simulink model "T10_LoNhiet"  (R2013b)
settings: Solver=ode5  StartTime=0.0  StopTime=inf  RelTol=1e-3
undefined symbols (not defined in the file or in its folder): National_Instruments, PCI
libraries: rtwinlib x4, dsparch4 x1, simulink x1
settings Model: SimulationMode=external  Creator=Administrator  LastModifiedBy=Administrator
settings HardwareCC: ProdIntDivRoundTo=Zero  ProdEndianess=LittleEndian  ProdHWDeviceType=Generic->32-bit x86 compatible
settings RTWCC: SystemTargetFile=rtwin.tlc  TemplateMakefile=rtwin.tmf  Description=Real-Time Windows Target  ProcessScript=rtwin_make_rtw_hook  RTWCompilerOptimization=On
settings CodeAppCC: MaxIdLength=95
settings RTWinTargetCC: TargetLibSuffix=_rtwin.lib  TargetPreCompLibLocation=C:\Program Files\MATLAB\R2013b\toolbox\rtw\targets\rtwin\lib\win64  CodeReplacementLibrary=ANSI_C  RTWinDir=C:/PROGRA~1/MATLAB/R2013b/toolbox/rtw/targets/rtwin  TargetArch=win64

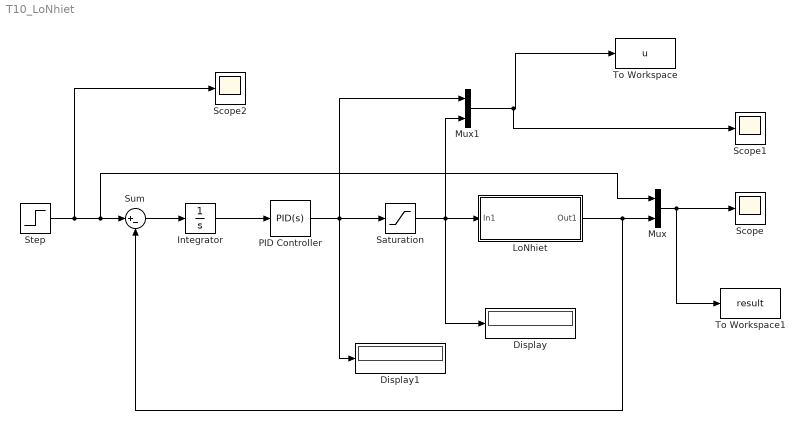
== system T10_LoNhiet ==
  Display : Display
  Display1 : Display
  Integrator : Integrator
  "LoNhiet " : Subsystem
  Mux : Mux  Inputs=2
  Mux1 : Mux  Inputs=2
  PID Controller : simulink/Continuous/PID Controller  Controller=PID  TimeDomain=Continuous-time  SampleTime=1  IntegratorMethod=Forward Euler  FilterMethod=Forward Euler  Form=Parallel  P=0.01  I=0.0005  D=0.0000025  N=100  InitialConditionSource=internal  InitialConditionForIntegrator=0  InitialConditionForFilter=0  ExternalReset=none  LimitOutput=off  UpperSaturationLimit=inf  LowerSaturationLimit=-inf  LinearizeAsGain=on  AntiWindupMode=none  Kb=1  TrackingMode=off  Kt=1  PParamMin=[]  PParamMax=[]  IParamMin=[]  IParamMax=[]  DParamMin=[]  DParamMax=[]  NParamMin=[]  NParamMax=[]  KbParamMin=[]  KbParamMax=[]  KtParamMin=[]  KtParamMax=[]  POutMin=[]  POutMax=[]  IOutMin=[]  IOutMax=[]  DOutMin=[]  DOutMax=[]  NOutMin=[]  NOutMax=[]  KbOutMin=[]  KbOutMax=[]  KtOutMin=[]  KtOutMax=[]  IntegratorOutMin=[]  IntegratorOutMax=[]  FilterOutMin=[]  FilterOutMax=[]  SumOutMin=[]  SumOutMax=[]  SumI1OutMin=[]  SumI1OutMax=[]  SumI2OutMin=[]  SumI2OutMax=[]  SumI3OutMin=[]  SumI3OutMax=[]  SumDOutMin=[]  SumDOutMax=[]  SaturationOutMin=[]  SaturationOutMax=[]  IntegratorContinuousStateAttributes=''  IntegratorStateMustResolveToSignalObject=off  IntegratorRTWStateStorageClass=Auto  FilterContinuousStateAttributes=''  FilterStateMustResolveToSignalObject=off  FilterRTWStateStorageClass=Auto
  Saturation : Saturate  UpperLimit=12  LowerLimit=0
  Scope : Scope
      settings: YMin=48  YMax=60
  Scope1 : Scope
      settings: YMin=0  YMax=2000
  Scope2 : Scope
      settings: YMin=60  YMax=60  SaveName=ScopeData2
  Step : Step  Time=0  After=60  SampleTime=0
  Sum : Sum  Inputs=|+-
  To Workspace : ToWorkspace  VariableName=u  SampleTime=-1  SaveFormat=Timeseries
  To Workspace1 : ToWorkspace  VariableName=result  SampleTime=-1  SaveFormat=Timeseries
  wires:
  Sum/1 -> Integrator/1
  Integrator/1 -> PID Controller/1
  PID Controller/1 -> Mux1/1, Display1/1, Saturation/1
  Saturation/1 -> Display/1, Mux1/2, "LoNhiet "/1(In1)
  Mux1/1 -> Scope1/1, To Workspace/1
  Mux/1 -> To Workspace1/1, Scope/1
  Step/1 -> Scope2/1, Mux/1, Sum/1
  "LoNhiet "/1(Out1) -> Sum/2, Mux/2

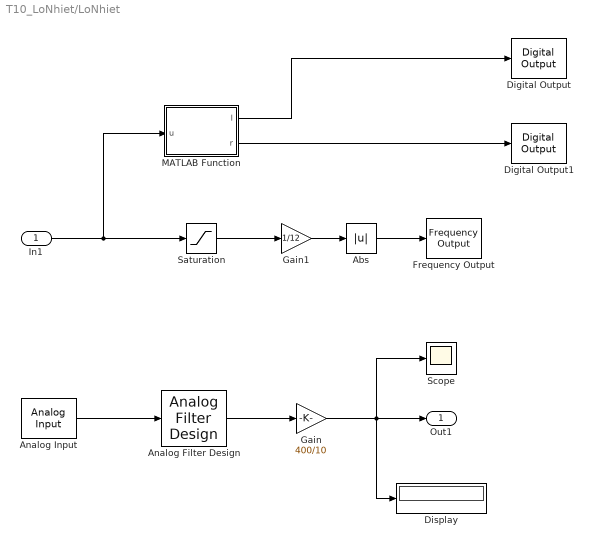
== system T10_LoNhiet/LoNhiet  ==
  In1 : Inport
  Abs : Abs
  Analog Filter Design : dsparch4/Analog Filter Design  method=Butterworth  filttype=Lowpass  N=4  Wlo=60  Whi=80  Rp=2  Rs=40
  Analog Input : rtwinlib/Analog Input  SampleTime=0.01  MaxMissedTicks=10  ShowMissedTicks=off  YieldWhenWaiting=off  DrvName=National_Instruments/PCI-6221  DrvAddress=4294967295  DrvOptions=[0 15 61600 2 3]  Channels=1  RangeMode=1  VoltRange=1  DataType=1
      settings: AttributesFormatString=National Instruments\nPCI-6221 [auto]
  Digital Output : rtwinlib/Digital Output  SampleTime=0.01  MaxMissedTicks=10  ShowMissedTicks=off  YieldWhenWaiting=off  DrvName=National_Instruments/PCI-6221  DrvAddress=4294967295  DrvOptions=[0 15 61600 2 3]  Channels=3  BitMode=1  InitialValue=[]  FinalValue=[]
      settings: AttributesFormatString=National Instruments\nPCI-6221 [auto]
  Digital Output1 : rtwinlib/Digital Output  SampleTime=0.01  MaxMissedTicks=10  ShowMissedTicks=off  YieldWhenWaiting=off  DrvName=National_Instruments/PCI-6221  DrvAddress=4294967295  DrvOptions=[0 15 61600 2 3]  Channels=4  BitMode=1  InitialValue=[]  FinalValue=[]
      settings: AttributesFormatString=National Instruments\nPCI-6221 [auto]
  Display : Display
  Frequency Output : rtwinlib/Frequency Output  SampleTime=0.01  MaxMissedTicks=10  ShowMissedTicks=off  YieldWhenWaiting=off  DrvName=National_Instruments/PCI-6221  DrvAddress=4294967295  DrvOptions=[0 15 61600 2 3]  Channels=2  FrequencySource=2  Frequency=[]  FrequencyFinalValue=[]  DutySource=1  Duty=0.5  DutyFinalValue=[]
      settings: AttributesFormatString=National Instruments\nPCI-6221 [auto]
  Gain : Gain  Gain=400/10
  Gain1 : Gain  Gain=1/12
  MATLAB Function : MATLAB Function  TreatAsAtomicUnit=on
  Saturation : Saturate  UpperLimit=12  LowerLimit=0
  Scope : Scope
      settings: SaveName=ScopeData3
  Out1 : Outport
  wires:
  Analog Input/1 -> Analog Filter Design/1
  Analog Filter Design/1 -> Gain/1
  Gain/1 -> Display/1, Scope/1, Out1/1
  In1/1 -> MATLAB Function/1(u), Saturation/1
  Saturation/1 -> Gain1/1
  Gain1/1 -> Abs/1
  MATLAB Function/1(l) -> Digital Output/1
  Abs/1 -> Frequency Output/1
  MATLAB Function/2(r) -> Digital Output1/1

== matlab function T10_LoNhiet/LoNhiet /MATLAB Function ==
  data: u input; l output; r output
function [l,r]=fcn(u)
if u>0
    l=1;
    r=0;
else
    l=0;
    r=0;
end
end
